simulink model "final_problema_4_sim"  (R2024b)
settings: Solver=VariableStepAuto  StartTime=0.0  StopTime=1000  RelTol=1e-3
values from neighbouring files (symbols this model uses):
  A = double(A)    [final_problema_3.m]    (also in final_problema_4.m = [-0.125000000000000,0.125000000000000,0.250000000000000)
  B = double(B)    [final_problema_3.m]    (also in final_problema_4.m = [0;0;0.020000000000000])
  C = k*(1/s)*((s+1)^2/(s+50)^2)    [final_problema_2.m]    (also in final_problema_3.m = k*(1/s)*(s+0.02)*(s+0.059)/(s+1.066); final_problema_4.m = [0 1 0])
  K = Ka(1:order(G))    [final_problema_4.m]
  kI = -Ka(end)    [final_problema_4.m]
settings Model: Creator=aghersin  LastModifiedBy=cgbri
settings SolverCC: AlgebraicLoopSolver=TrustRegion
settings DataIOCC: ReturnWorkspaceOutputs=off
settings DebuggingCC: UnconnectedInputMsg=warning  UnconnectedOutputMsg=warning  UnconnectedLineMsg=warning  ArithmeticOperatorsInVariantConditions=warning
settings ModelReferenceCC: EnableRefExpFcnMdlSchedulingChecks=on
settings SFSimCC: SimUseLocalCustomCode=off  CustomCodeUndefinedFunction=UseInterfaceOnly
settings RTWCC: RTWUseLocalCustomCode=off  GPUComputeCapability=3.5

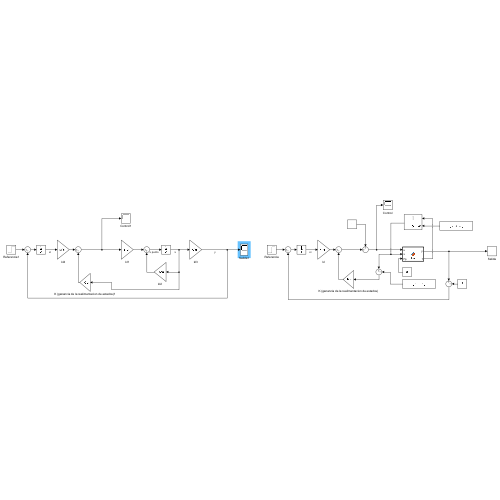
[thumbnail: Simulink's stored preview of the top-level diagram]
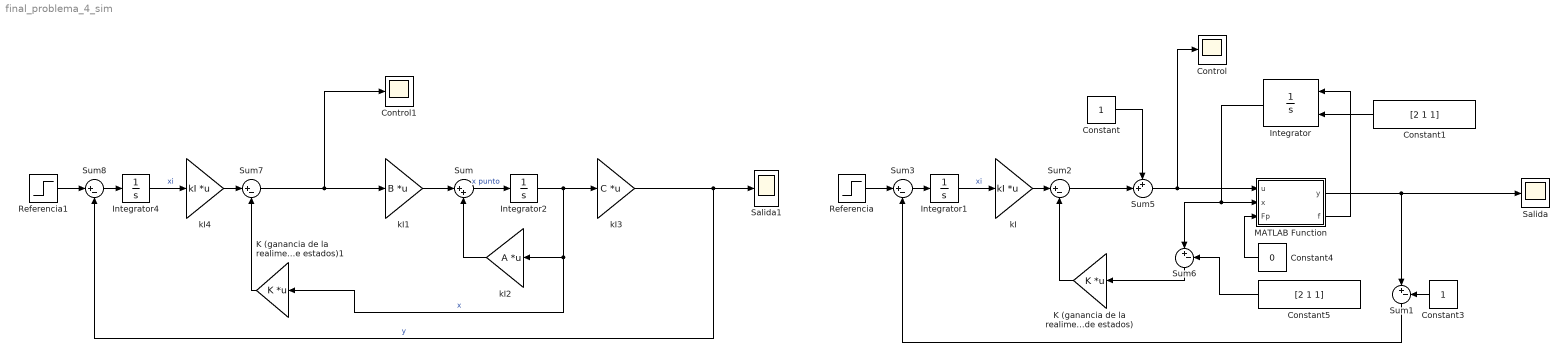
== system final_problema_4_sim ==
  Constant : Constant
  Constant1 : Constant  Value=[2 1 1]
  Constant3 : Constant
  Constant4 : Constant  Value=0
  Constant5 : Constant  Value=[2 1 1]
  Control : Scope
  Control1 : Scope
  Integrator : Integrator  InitialConditionSource=external
  Integrator1 : Integrator
  Integrator2 : Integrator
  Integrator4 : Integrator
  K (ganancia de la realimentacion de estados) : Gain  Gain=K  Multiplication=Matrix(K*u)
  K (ganancia de la realimentacion de estados)1 : Gain  Gain=K  Multiplication=Matrix(K*u)
  MATLAB Function : MATLAB Function  TreatAsAtomicUnit=on
  Referencia : Step  After=0.1  SampleTime=0
  Referencia1 : Step  After=0.1  SampleTime=0
  Salida : Scope
  Salida1 : Scope
  Sum : Sum  Inputs=|++
  Sum{1..3,6..8} (6 alike) : Sum  Inputs=|+-
  Sum5 : Sum  Inputs=++|
  kI : Gain  Gain=kI  Multiplication=Matrix(K*u)
  kI1 : Gain  Gain=B  Multiplication=Matrix(K*u)
  kI2 : Gain  Gain=A  Multiplication=Matrix(K*u)
  kI3 : Gain  Gain=C  Multiplication=Matrix(K*u)
  kI4 : Gain  Gain=kI  Multiplication=Matrix(K*u)
  wires:
  Referencia/1 -> Sum3/1
  Sum3/1 -> Integrator1/1
  K (ganancia de la realimentacion de estados)/1 -> Sum2/2
  kI/1 -> Sum2/1
  Integrator1/1 -> kI/1  "xi"
  MATLAB Function/1(y) -> Salida/1, Sum1/1
  Constant3/1 -> Sum1/2
  Constant1/1 -> Integrator/2
  MATLAB Function/2(f) -> Integrator/1
  Integrator/1 -> Sum6/1, MATLAB Function/2(x)
  Constant4/1 -> MATLAB Function/3(Fp)
  Sum2/1 -> Sum5/2
  Sum1/1 -> Sum3/2
  Sum6/1 -> K (ganancia de la realimentacion de estados)/1
  Constant5/1 -> Sum6/2
  Sum5/1 -> Control/1, MATLAB Function/1(u)
  Constant/1 -> Sum5/1
  Integrator2/1 -> kI3/1, K (ganancia de la realimentacion de estados)1/1, kI2/1  "x"
  kI2/1 -> Sum/2
  kI1/1 -> Sum/1
  Sum/1 -> Integrator2/1  "x punto"
  kI3/1 -> Salida1/1, Sum8/2  "y"
  Sum8/1 -> Integrator4/1
  Referencia1/1 -> Sum8/1
  kI4/1 -> Sum7/1
  Integrator4/1 -> kI4/1  "xi"
  K (ganancia de la realimentacion de estados)1/1 -> Sum7/2
  Sum7/1 -> Control1/1, kI1/1

== matlab function final_problema_4_sim/MATLAB Function ==
  data: u input; y output; x input; f output; Fp input
function [y,f] = fcn(u, x, Fp)
    %Constantes
    p = 0.02;
    
    %Ecuaciones no lineales
    F1 = ( x(3) - sqrt(abs(x(1)-x(2))) )/power(x(1), 2);
    F2 = ( sqrt(abs(x(1)-x(2))) - sqrt(abs(x(2))) + Fp )/power(x(2), 2);
    F3 = p*u-p*x(3);
    
    y = x(2);
    f = [F1 F2 F3];
